simulink model "lab1"  (R2020b)
settings: Solver=VariableStepAuto  StartTime=0.0  StopTime=10.0  RelTol=1e-3
libraries: powerlib x8, simulink x1
settings Model: Creator=hp  LastModifiedBy=Lenovo

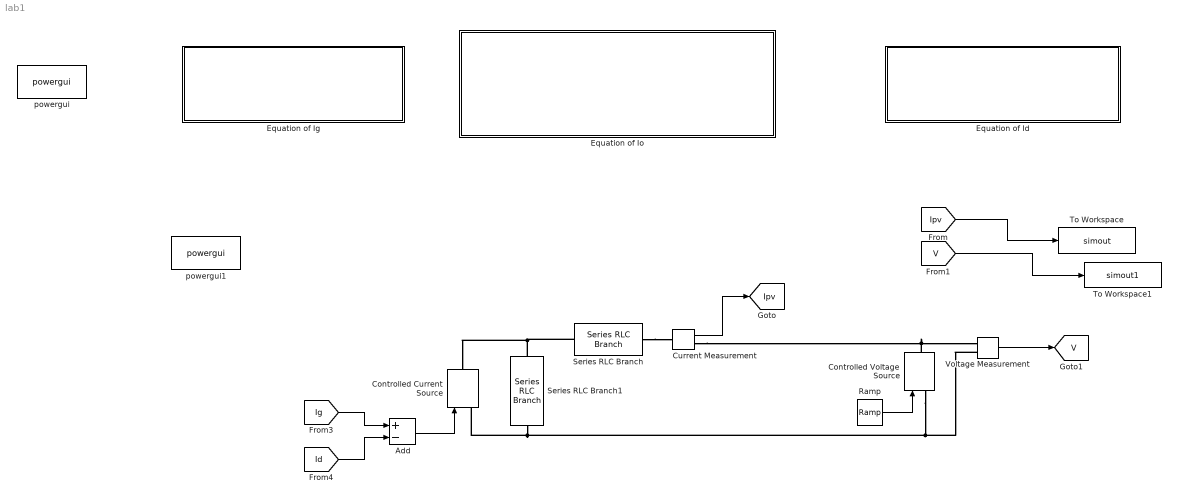
== system lab1 ==
  Add : Sum  Inputs=+-
  Controlled Current Source : powerlib/Electrical Sources/Controlled Current Source  Initialize=on  Source_Type=AC  Amplitude=0  Phase=0  Frequency=0  Measurements=None
  Controlled Voltage Source : powerlib/Electrical Sources/Controlled Voltage Source  Initialize=on  Source_Type=AC  Amplitude=0  Phase=0  Frequency=0  Measurements=None
  Current Measurement : powerlib/Measurements/Current Measurement  PhasorSimulation=off  OutputType=Complex  PSBequivalent=0
  Equation of Id : Subsystem
  Equation of Ig : Subsystem
  Equation of Io : Subsystem
  Ramp : simulink/Sources/Ramp  slope=3.29  start=0  InitialOutput=0
  Series RLC Branch : powerlib/Elements/Series RLC Branch  LConnTagsString=__new0  RConnTagsString=__new0  BranchType=R  Resistance=0.221  Inductance=1e-3  SetiL0=off  InitialCurrent=0  Capacitance=1e-6  Setx0=off  InitialVoltage=0  Measurements=None
  Series RLC Branch1 : powerlib/Elements/Series RLC Branch  LConnTagsString=__new0  RConnTagsString=__new0  BranchType=R  Resistance=414.5  Inductance=1e-3  SetiL0=off  InitialCurrent=0  Capacitance=1e-6  Setx0=off  InitialVoltage=0  Measurements=None
  To Workspace : ToWorkspace  VariableName=simout  SaveFormat=Timeseries  SampleTime=-1
  To Workspace1 : ToWorkspace  VariableName=simout1  SaveFormat=Timeseries  SampleTime=-1
  Voltage Measurement : powerlib/Measurements/Voltage Measurement  PhasorSimulation=off  OutputType=Complex  PSBequivalent=0
  powergui : powerlib/powergui  Priority=1  SimulationMode=Discrete  SampleTime=50e-6  frequency=60  Iterations=50  frequencyindice=0  Pbase=100e6  ErrMax=1e-4  UnitsV=kV  UnitsW=MW  buscounter=0  FunctionMessages=off  echomessages=off  EnableUseOfTLC=off  CurrentSourceSwitches=off  DisableSnubberDevices=off  DisableRonSwitches=off  DisableVfSwitches=off  DisplayEquations=off  AutomaticDiscreteSolvers=off  SolverType=Tustin/Backward Euler (TBE)  Interpol=off  ExternalGateDelay=off  methode=off  Ts=100  x0status=blocks  SPID=on  SwTol=0  HookPort=off  NonlinearTolerance=1e-4  nMaxIteration=100  ContinueOnMaxIteration=off  RestoreLinks=warning  ResistiveCurrentMeasurement=off  Frange=[0:2:500]  Ylog=off  Xlog=on  ShowGrid=off  save=off  variable=ZData  structure=0  ZoomFFT=off  StartTime=0.0  cycles=1  DisplayStyle=1  fundamental=60  FreqAxis=off  MaxFrequency=1000  frequencyindicesteady=1  RmsSteady=1  display=off
  powergui1 : powerlib/powergui  Priority=1  SimulationMode=Continuous  SampleTime=50e-6  frequency=60  Iterations=50  frequencyindice=60  Pbase=100e6  ErrMax=1e-4  UnitsV=kV  UnitsW=MW  buscounter=0  FunctionMessages=off  echomessages=off  EnableUseOfTLC=off  CurrentSourceSwitches=off  DisableSnubberDevices=off  DisableRonSwitches=off  DisableVfSwitches=off  DisplayEquations=off  AutomaticDiscreteSolvers=off  SolverType=Tustin/Backward Euler (TBE)  Interpol=off  ExternalGateDelay=off  methode=off  Ts=100  x0status=blocks  SPID=on  SwTol=0  HookPort=off  NonlinearTolerance=1e-4  nMaxIteration=100  ContinueOnMaxIteration=off  RestoreLinks=warning  ResistiveCurrentMeasurement=off  Frange=[0:2:500]  Ylog=off  Xlog=on  ShowGrid=off  save=off  variable=ZData  structure=0  ZoomFFT=off  StartTime=0.0  cycles=1  DisplayStyle=1  fundamental=60  FreqAxis=off  MaxFrequency=1000  frequencyindicesteady=1  RmsSteady=1  display=off
  tag scope: Ipv=global, V=global
  wires:
  [Ig] -> Add/1
  [Id] -> Add/2
  Add/1 -> Controlled Current Source/1
  Ramp/1 -> Controlled Voltage Source/1
  Voltage Measurement/1 -> [V]
  [Ipv] -> To Workspace/1
  [V] -> To Workspace1/1
  Current Measurement/1 -> [Ipv]
  connections:
  Controlled Voltage Source/LConn1 -- Voltage Measurement/LConn2 -- Series RLC Branch1/RConn1 -- Controlled Current Source/LConn1
  Current Measurement/RConn1 -- Controlled Voltage Source/RConn1 -- Voltage Measurement/LConn1
  Series RLC Branch1/LConn1 -- Series RLC Branch/LConn1 -- Controlled Current Source/RConn1
  Series RLC Branch/RConn1 -- Current Measurement/LConn1

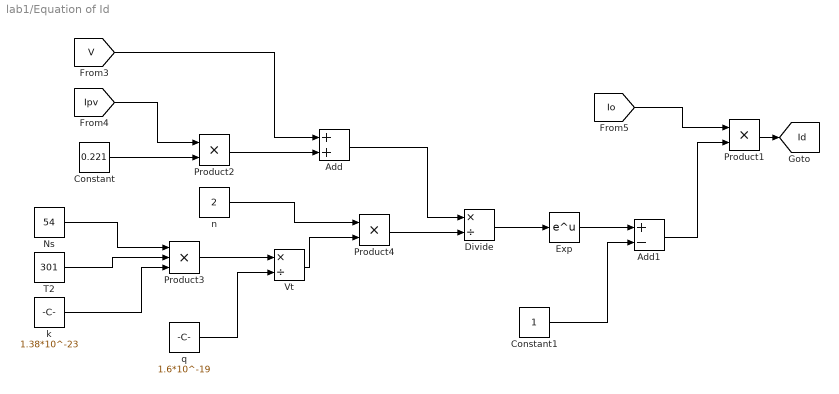
== system lab1/Equation of Id ==
  Add : Sum
  Add1 : Sum  Inputs=+-
  Constant : Constant  Value=0.221
  Constant1 : Constant
  Divide : Product  Inputs=*/
  Exp : Math  SaturateOnIntegerOverflow=on
  Ns : Constant  Value=54
  Product1 : Product
  Product2 : Product
  Product3 : Product  Inputs=3
  Product4 : Product
  T2 : Constant  Value=301
  Vt : Product  Inputs=*/
  k : Constant  Value=1.38*10^-23
  n : Constant  Value=2
  q : Constant  Value=1.6*10^-19
  tag scope: Id=global
  wires:
  k/1 -> Product3/3
  Ns/1 -> Product3/1
  T2/1 -> Product3/2
  Vt/1 -> Product4/2
  Constant1/1 -> Add1/2
  q/1 -> Vt/2
  n/1 -> Product4/1
  Product3/1 -> Vt/1
  Constant/1 -> Product2/2
  Product4/1 -> Divide/2
  [V] -> Add/1
  Add1/1 -> Product1/2
  Divide/1 -> Exp/1
  [Io] -> Product1/1
  Exp/1 -> Add1/1
  Product2/1 -> Add/2
  [Ipv] -> Product2/1
  Product1/1 -> [Id]
  Add/1 -> Divide/1

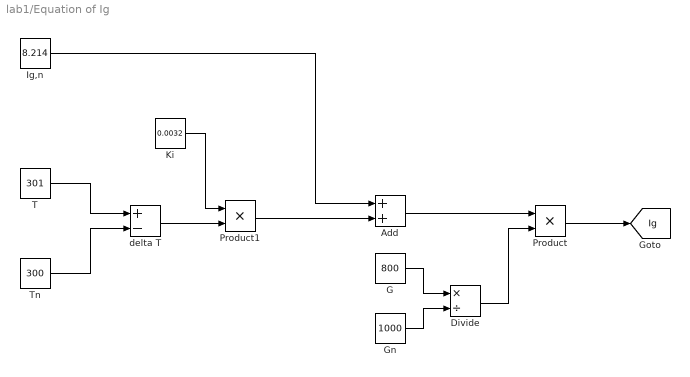
== system lab1/Equation of Ig ==
  Add : Sum
  Divide : Product  Inputs=*/
  G : Constant  Value=800
  Gn : Constant  Value=1000
  Ig,n : Constant  Value=8.214
  Ki : Constant  Value=0.0032
  Product : Product
  Product1 : Product
  T : Constant  Value=301
  Tn : Constant  Value=300
  delta T : Sum  Inputs=+-
  tag scope: Ig=global
  wires:
  Gn/1 -> Divide/2
  Add/1 -> Product/1
  Product1/1 -> Add/2
  G/1 -> Divide/1
  delta T/1 -> Product1/2
  T/1 -> delta T/1
  Ki/1 -> Product1/1
  Tn/1 -> delta T/2
  Ig,n/1 -> Add/1
  Divide/1 -> Product/2
  Product/1 -> [Ig]

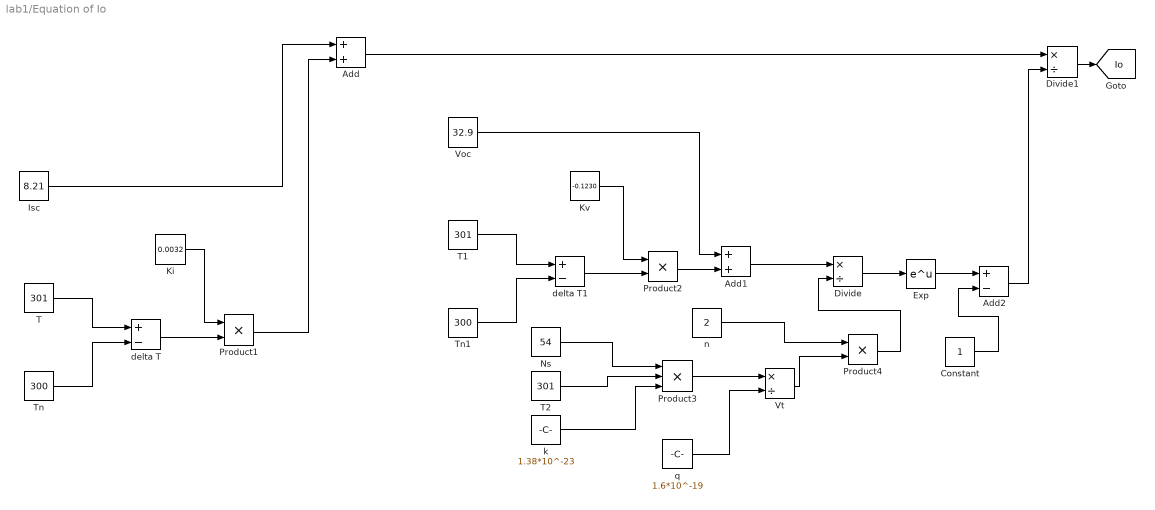
== system lab1/Equation of Io ==
  Add : Sum
  Add1 : Sum
  Add2 : Sum  Inputs=+-
  Constant : Constant
  Divide : Product  Inputs=*/
  Divide1 : Product  Inputs=*/
  Exp : Math  SaturateOnIntegerOverflow=on
  Isc : Constant  Value=8.21
  Ki : Constant  Value=0.0032
  Kv : Constant  Value=-0.1230
  Ns : Constant  Value=54
  Product1 : Product
  Product2 : Product
  Product3 : Product  Inputs=3
  Product4 : Product
  T : Constant  Value=301
  T1 : Constant  Value=301
  T2 : Constant  Value=301
  Tn : Constant  Value=300
  Tn1 : Constant  Value=300
  Voc : Constant  Value=32.9
  Vt : Product  Inputs=*/
  delta T : Sum  Inputs=+-
  delta T1 : Sum  Inputs=+-
  k : Constant  Value=1.38*10^-23
  n : Constant  Value=2
  q : Constant  Value=1.6*10^-19
  tag scope: Io=global
  wires:
  Isc/1 -> Add/1
  Kv/1 -> Product2/1
  Exp/1 -> Add2/1
  Constant/1 -> Add2/2
  k/1 -> Product3/3
  Product3/1 -> Vt/1
  Add1/1 -> Divide/1
  Tn1/1 -> delta T1/2
  Tn/1 -> delta T/2
  Product4/1 -> Divide/2
  Ns/1 -> Product3/1
  T2/1 -> Product3/2
  Voc/1 -> Add1/1
  Vt/1 -> Product4/2
  Product2/1 -> Add1/2
  q/1 -> Vt/2
  n/1 -> Product4/1
  Divide/1 -> Exp/1
  Product1/1 -> Add/2
  delta T1/1 -> Product2/2
  T/1 -> delta T/1
  Ki/1 -> Product1/1
  Add2/1 -> Divide1/2
  delta T/1 -> Product1/2
  T1/1 -> delta T1/1
  Add/1 -> Divide1/1
  Divide1/1 -> [Io]
